simulink model "r17_27"  (Simulink 8.6)
settings: Solver=FixedStepDiscrete  StartTime=0.0  StopTime=500  FixedStep=0.1  RelTol=1e-3
undefined symbols (not defined in the file or in its folder): sldvsubsys
libraries: sldvlib x16, simulink x12
(part 2 of 2)

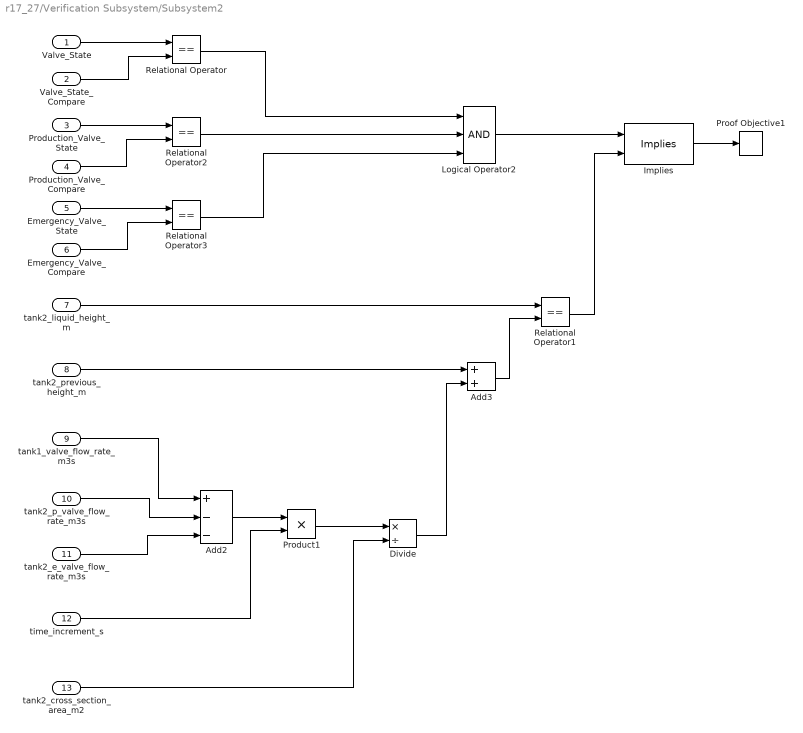
== system r17_27/Verification Subsystem/Subsystem2 ==
  Valve_State : Inport
  Valve_State_Compare : Inport  Port=2
  Production_Valve_State : Inport  Port=3
  Production_Valve_Compare : Inport  Port=4
  Emergency_Valve_State : Inport  Port=5
  Emergency_Valve_Compare : Inport  Port=6
  tank2_liquid_height_m : Inport  Port=7
  tank2_previous_height_m : Inport  Port=8
  tank1_valve_flow_rate_m3s : Inport  Port=9
  tank2_p_valve_flow_rate_m3s : Inport  Port=10
  tank2_e_valve_flow_rate_m3s : Inport  Port=11
  time_increment_s : Inport  Port=12
  tank2_cross_section_area_m2 : Inport  Port=13
  Add2 : Sum  Inputs=+--
  Add3 : Sum
  Divide : Product  Inputs=*/
  Implies : sldvlib/Verification Utilities/Implies
  Logical Operator2 : Logic  Inputs=3  AllPortsSameDT=off  OutDataTypeStr=boolean
  Product1 : Product
  Proof Objective1 : sldvlib/Objectives and Constraints/Proof Objective  enabled=on  customAVTBlockType=Proof Objective  intervals=true  dispValues=on  outEnabled=off  enableStopSim=off
      settings: AttributesFormatString=%<intervals>
  Relational Operator{,1..3} (4 alike) : RelationalOperator  Operator===  OutDataTypeStr=boolean
  wires:
  Valve_State/1 -> Relational Operator/1
  Relational Operator1/1 -> Implies/2
  Add2/1 -> Product1/1
  tank2_cross_section_area_m2/1 -> Divide/2
  Add3/1 -> Relational Operator1/2
  Logical Operator2/1 -> Implies/1
  Product1/1 -> Divide/1
  tank2_previous_height_m/1 -> Add3/1
  tank1_valve_flow_rate_m3s/1 -> Add2/1
  tank2_e_valve_flow_rate_m3s/1 -> Add2/3
  Relational Operator3/1 -> Logical Operator2/3
  time_increment_s/1 -> Product1/2
  Relational Operator2/1 -> Logical Operator2/2
  Emergency_Valve_State/1 -> Relational Operator3/1
  tank2_p_valve_flow_rate_m3s/1 -> Add2/2
  tank2_liquid_height_m/1 -> Relational Operator1/1
  Divide/1 -> Add3/2
  Production_Valve_State/1 -> Relational Operator2/1
  Implies/1 -> Proof Objective1/1
  Valve_State_Compare/1 -> Relational Operator/2
  Emergency_Valve_Compare/1 -> Relational Operator3/2
  Production_Valve_Compare/1 -> Relational Operator2/2
  Relational Operator/1 -> Logical Operator2/1

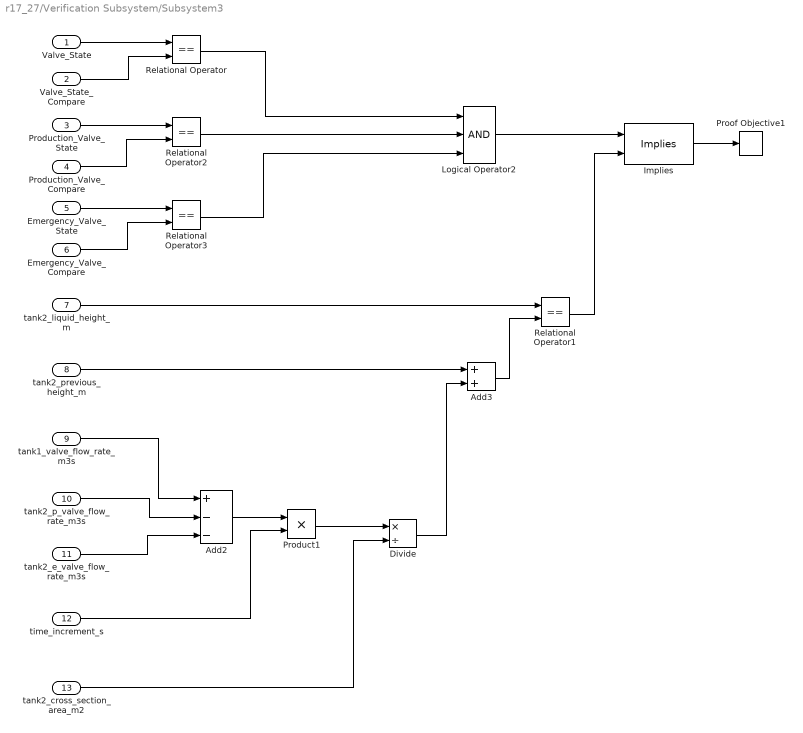
== system r17_27/Verification Subsystem/Subsystem3 ==
  Valve_State : Inport
  Valve_State_Compare : Inport  Port=2
  Production_Valve_State : Inport  Port=3
  Production_Valve_Compare : Inport  Port=4
  Emergency_Valve_State : Inport  Port=5
  Emergency_Valve_Compare : Inport  Port=6
  tank2_liquid_height_m : Inport  Port=7
  tank2_previous_height_m : Inport  Port=8
  tank1_valve_flow_rate_m3s : Inport  Port=9
  tank2_p_valve_flow_rate_m3s : Inport  Port=10
  tank2_e_valve_flow_rate_m3s : Inport  Port=11
  time_increment_s : Inport  Port=12
  tank2_cross_section_area_m2 : Inport  Port=13
  Add2 : Sum  Inputs=+--
  Add3 : Sum
  Divide : Product  Inputs=*/
  Implies : sldvlib/Verification Utilities/Implies
  Logical Operator2 : Logic  Inputs=3  AllPortsSameDT=off  OutDataTypeStr=boolean
  Product1 : Product
  Proof Objective1 : sldvlib/Objectives and Constraints/Proof Objective  enabled=on  customAVTBlockType=Proof Objective  intervals=true  dispValues=on  outEnabled=off  enableStopSim=off
      settings: AttributesFormatString=%<intervals>
  Relational Operator{,1..3} (4 alike) : RelationalOperator  Operator===  OutDataTypeStr=boolean
  wires:
  Valve_State/1 -> Relational Operator/1
  Relational Operator1/1 -> Implies/2
  Add2/1 -> Product1/1
  tank2_cross_section_area_m2/1 -> Divide/2
  Add3/1 -> Relational Operator1/2
  Logical Operator2/1 -> Implies/1
  Product1/1 -> Divide/1
  tank2_previous_height_m/1 -> Add3/1
  tank1_valve_flow_rate_m3s/1 -> Add2/1
  tank2_e_valve_flow_rate_m3s/1 -> Add2/3
  Relational Operator3/1 -> Logical Operator2/3
  time_increment_s/1 -> Product1/2
  Relational Operator2/1 -> Logical Operator2/2
  Emergency_Valve_State/1 -> Relational Operator3/1
  tank2_p_valve_flow_rate_m3s/1 -> Add2/2
  tank2_liquid_height_m/1 -> Relational Operator1/1
  Divide/1 -> Add3/2
  Production_Valve_State/1 -> Relational Operator2/1
  Implies/1 -> Proof Objective1/1
  Valve_State_Compare/1 -> Relational Operator/2
  Emergency_Valve_Compare/1 -> Relational Operator3/2
  Production_Valve_Compare/1 -> Relational Operator2/2
  Relational Operator/1 -> Logical Operator2/1

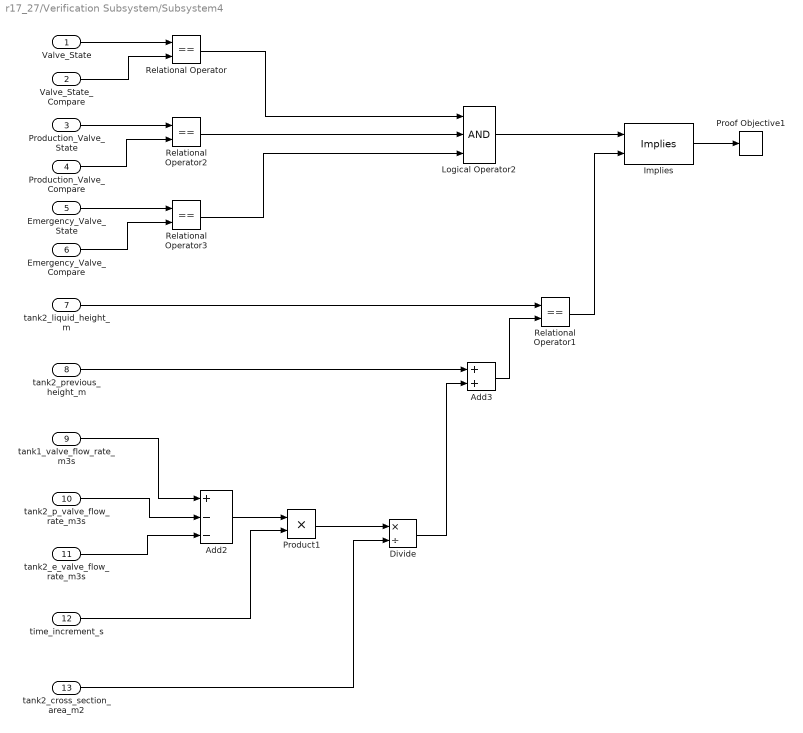
== system r17_27/Verification Subsystem/Subsystem4 ==
  Valve_State : Inport
  Valve_State_Compare : Inport  Port=2
  Production_Valve_State : Inport  Port=3
  Production_Valve_Compare : Inport  Port=4
  Emergency_Valve_State : Inport  Port=5
  Emergency_Valve_Compare : Inport  Port=6
  tank2_liquid_height_m : Inport  Port=7
  tank2_previous_height_m : Inport  Port=8
  tank1_valve_flow_rate_m3s : Inport  Port=9
  tank2_p_valve_flow_rate_m3s : Inport  Port=10
  tank2_e_valve_flow_rate_m3s : Inport  Port=11
  time_increment_s : Inport  Port=12
  tank2_cross_section_area_m2 : Inport  Port=13
  Add2 : Sum  Inputs=+--
  Add3 : Sum
  Divide : Product  Inputs=*/
  Implies : sldvlib/Verification Utilities/Implies
  Logical Operator2 : Logic  Inputs=3  AllPortsSameDT=off  OutDataTypeStr=boolean
  Product1 : Product
  Proof Objective1 : sldvlib/Objectives and Constraints/Proof Objective  enabled=on  customAVTBlockType=Proof Objective  intervals=true  dispValues=on  outEnabled=off  enableStopSim=off
      settings: AttributesFormatString=%<intervals>
  Relational Operator{,1..3} (4 alike) : RelationalOperator  Operator===  OutDataTypeStr=boolean
  wires:
  Valve_State/1 -> Relational Operator/1
  Relational Operator1/1 -> Implies/2
  Add2/1 -> Product1/1
  tank2_cross_section_area_m2/1 -> Divide/2
  Add3/1 -> Relational Operator1/2
  Logical Operator2/1 -> Implies/1
  Product1/1 -> Divide/1
  tank2_previous_height_m/1 -> Add3/1
  tank1_valve_flow_rate_m3s/1 -> Add2/1
  tank2_e_valve_flow_rate_m3s/1 -> Add2/3
  Relational Operator3/1 -> Logical Operator2/3
  time_increment_s/1 -> Product1/2
  Relational Operator2/1 -> Logical Operator2/2
  Emergency_Valve_State/1 -> Relational Operator3/1
  tank2_p_valve_flow_rate_m3s/1 -> Add2/2
  tank2_liquid_height_m/1 -> Relational Operator1/1
  Divide/1 -> Add3/2
  Production_Valve_State/1 -> Relational Operator2/1
  Implies/1 -> Proof Objective1/1
  Valve_State_Compare/1 -> Relational Operator/2
  Emergency_Valve_Compare/1 -> Relational Operator3/2
  Production_Valve_Compare/1 -> Relational Operator2/2
  Relational Operator/1 -> Logical Operator2/1

== system r17_27/Verification Subsystem/Subsystem5 ==
  Valve_State : Inport
  Valve_State_Compare : Inport  Port=2
  Production_Valve_State : Inport  Port=3
  Production_Valve_Compare : Inport  Port=4
  Emergency_Valve_State : Inport  Port=5
  Emergency_Valve_Compare : Inport  Port=6
  tank2_liquid_height_m : Inport  Port=7
  tank2_previous_height_m : Inport  Port=8
  tank1_valve_flow_rate_m3s : Inport  Port=9
  tank2_p_valve_flow_rate_m3s : Inport  Port=10
  tank2_e_valve_flow_rate_m3s : Inport  Port=11
  time_increment_s : Inport  Port=12
  tank2_cross_section_area_m2 : Inport  Port=13
  Add2 : Sum  Inputs=+--
  Add3 : Sum
  Divide : Product  Inputs=*/
  Implies : sldvlib/Verification Utilities/Implies
  Logical Operator2 : Logic  Inputs=3  AllPortsSameDT=off  OutDataTypeStr=boolean
  Product1 : Product
  Proof Objective1 : sldvlib/Objectives and Constraints/Proof Objective  enabled=on  customAVTBlockType=Proof Objective  intervals=true  dispValues=on  outEnabled=off  enableStopSim=off
      settings: AttributesFormatString=%<intervals>
  Relational Operator{,1..3} (4 alike) : RelationalOperator  Operator===  OutDataTypeStr=boolean
  wires:
  Valve_State/1 -> Relational Operator/1
  Relational Operator1/1 -> Implies/2
  Add2/1 -> Product1/1
  tank2_cross_section_area_m2/1 -> Divide/2
  Add3/1 -> Relational Operator1/2
  Logical Operator2/1 -> Implies/1
  Product1/1 -> Divide/1
  tank2_previous_height_m/1 -> Add3/1
  tank1_valve_flow_rate_m3s/1 -> Add2/1
  tank2_e_valve_flow_rate_m3s/1 -> Add2/3
  Relational Operator3/1 -> Logical Operator2/3
  time_increment_s/1 -> Product1/2
  Relational Operator2/1 -> Logical Operator2/2
  Emergency_Valve_State/1 -> Relational Operator3/1
  tank2_p_valve_flow_rate_m3s/1 -> Add2/2
  tank2_liquid_height_m/1 -> Relational Operator1/1
  Divide/1 -> Add3/2
  Production_Valve_State/1 -> Relational Operator2/1
  Implies/1 -> Proof Objective1/1
  Valve_State_Compare/1 -> Relational Operator/2
  Emergency_Valve_Compare/1 -> Relational Operator3/2
  Production_Valve_Compare/1 -> Relational Operator2/2
  Relational Operator/1 -> Logical Operator2/1

== system r17_27/Verification Subsystem/Subsystem6 ==
  Valve_State : Inport
  Valve_State_Compare : Inport  Port=2
  Production_Valve_State : Inport  Port=3
  Production_Valve_Compare : Inport  Port=4
  Emergency_Valve_State : Inport  Port=5
  Emergency_Valve_Compare : Inport  Port=6
  tank2_liquid_height_m : Inport  Port=7
  tank2_previous_height_m : Inport  Port=8
  tank1_valve_flow_rate_m3s : Inport  Port=9
  tank2_p_valve_flow_rate_m3s : Inport  Port=10
  tank2_e_valve_flow_rate_m3s : Inport  Port=11
  time_increment_s : Inport  Port=12
  tank2_cross_section_area_m2 : Inport  Port=13
  Add2 : Sum  Inputs=+--
  Add3 : Sum
  Divide : Product  Inputs=*/
  Implies : sldvlib/Verification Utilities/Implies
  Logical Operator2 : Logic  Inputs=3  AllPortsSameDT=off  OutDataTypeStr=boolean
  Product1 : Product
  Proof Objective1 : sldvlib/Objectives and Constraints/Proof Objective  enabled=on  customAVTBlockType=Proof Objective  intervals=true  dispValues=on  outEnabled=off  enableStopSim=off
      settings: AttributesFormatString=%<intervals>
  Relational Operator{,1..3} (4 alike) : RelationalOperator  Operator===  OutDataTypeStr=boolean
  wires:
  Valve_State/1 -> Relational Operator/1
  Relational Operator1/1 -> Implies/2
  Add2/1 -> Product1/1
  tank2_cross_section_area_m2/1 -> Divide/2
  Add3/1 -> Relational Operator1/2
  Logical Operator2/1 -> Implies/1
  Product1/1 -> Divide/1
  tank2_previous_height_m/1 -> Add3/1
  tank1_valve_flow_rate_m3s/1 -> Add2/1
  tank2_e_valve_flow_rate_m3s/1 -> Add2/3
  Relational Operator3/1 -> Logical Operator2/3
  time_increment_s/1 -> Product1/2
  Relational Operator2/1 -> Logical Operator2/2
  Emergency_Valve_State/1 -> Relational Operator3/1
  tank2_p_valve_flow_rate_m3s/1 -> Add2/2
  tank2_liquid_height_m/1 -> Relational Operator1/1
  Divide/1 -> Add3/2
  Production_Valve_State/1 -> Relational Operator2/1
  Implies/1 -> Proof Objective1/1
  Valve_State_Compare/1 -> Relational Operator/2
  Emergency_Valve_Compare/1 -> Relational Operator3/2
  Production_Valve_Compare/1 -> Relational Operator2/2
  Relational Operator/1 -> Logical Operator2/1

== system r17_27/Verification Subsystem/Subsystem7 ==
  Valve_State : Inport
  Valve_State_Compare : Inport  Port=2
  Production_Valve_State : Inport  Port=3
  Production_Valve_Compare : Inport  Port=4
  Emergency_Valve_State : Inport  Port=5
  Emergency_Valve_Compare : Inport  Port=6
  tank2_liquid_height_m : Inport  Port=7
  tank2_previous_height_m : Inport  Port=8
  tank1_valve_flow_rate_m3s : Inport  Port=9
  tank2_p_valve_flow_rate_m3s : Inport  Port=10
  tank2_e_valve_flow_rate_m3s : Inport  Port=11
  time_increment_s : Inport  Port=12
  tank2_cross_section_area_m2 : Inport  Port=13
  Add2 : Sum  Inputs=+--
  Add3 : Sum
  Divide : Product  Inputs=*/
  Implies : sldvlib/Verification Utilities/Implies
  Logical Operator2 : Logic  Inputs=3  AllPortsSameDT=off  OutDataTypeStr=boolean
  Product1 : Product
  Proof Objective1 : sldvlib/Objectives and Constraints/Proof Objective  enabled=on  customAVTBlockType=Proof Objective  intervals=true  dispValues=on  outEnabled=off  enableStopSim=off
      settings: AttributesFormatString=%<intervals>
  Relational Operator{,1..3} (4 alike) : RelationalOperator  Operator===  OutDataTypeStr=boolean
  wires:
  Valve_State/1 -> Relational Operator/1
  Relational Operator1/1 -> Implies/2
  Add2/1 -> Product1/1
  tank2_cross_section_area_m2/1 -> Divide/2
  Add3/1 -> Relational Operator1/2
  Logical Operator2/1 -> Implies/1
  Product1/1 -> Divide/1
  tank2_previous_height_m/1 -> Add3/1
  tank1_valve_flow_rate_m3s/1 -> Add2/1
  tank2_e_valve_flow_rate_m3s/1 -> Add2/3
  Relational Operator3/1 -> Logical Operator2/3
  time_increment_s/1 -> Product1/2
  Relational Operator2/1 -> Logical Operator2/2
  Emergency_Valve_State/1 -> Relational Operator3/1
  tank2_p_valve_flow_rate_m3s/1 -> Add2/2
  tank2_liquid_height_m/1 -> Relational Operator1/1
  Divide/1 -> Add3/2
  Production_Valve_State/1 -> Relational Operator2/1
  Implies/1 -> Proof Objective1/1
  Valve_State_Compare/1 -> Relational Operator/2
  Emergency_Valve_Compare/1 -> Relational Operator3/2
  Production_Valve_Compare/1 -> Relational Operator2/2
  Relational Operator/1 -> Logical Operator2/1
